simulink model "Filter_Model"  (R2020b)
settings: Solver=VariableStepAuto  StartTime=0.0  StopTime=10.0  RelTol=1e-3
settings Model: Creator=BIDITA PAUL  LastModifiedBy=BIDITA PAUL

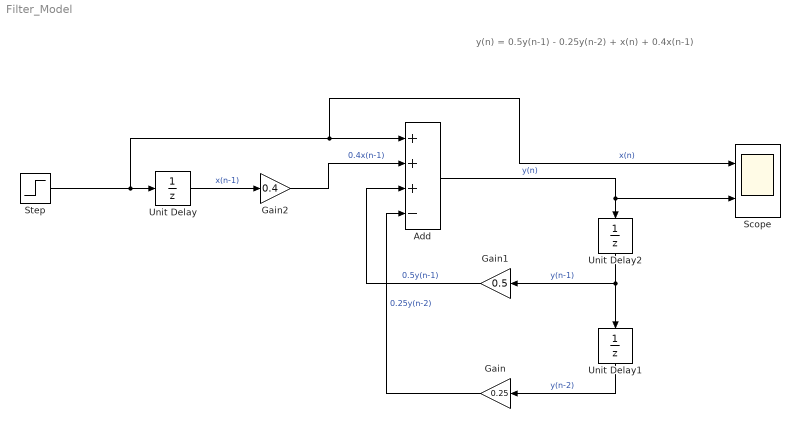
== system Filter_Model ==
  note: y(n) = 0.5y(n-1) - 0.25y(n-2) + x(n) + 0.4x(n-1)
  Add : Sum  Inputs=+++-
  Gain : Gain  Gain=0.25
  Gain1 : Gain  Gain=0.5
  Gain2 : Gain  Gain=0.4
  Scope : Scope  NumInputPorts=2
  Step : Step  SampleTime=0
  Unit Delay : UnitDelay  SampleTime=-1  HasFrameUpgradeWarning=on
  Unit Delay1 : UnitDelay  SampleTime=-1  HasFrameUpgradeWarning=on
  Unit Delay2 : UnitDelay  SampleTime=-1  HasFrameUpgradeWarning=on
  wires:
  Step/1 -> Add/1, Scope/1, Unit Delay/1  "x(n)"
  Unit Delay/1 -> Gain2/1  "x(n-1)"
  Add/1 -> Unit Delay2/1, Scope/2  "y(n)"
  Unit Delay2/1 -> Unit Delay1/1, Gain1/1  "y(n-1)"
  Unit Delay1/1 -> Gain/1  "y(n-2)"
  Gain/1 -> Add/4  "0.25y(n-2)"
  Gain1/1 -> Add/3  "0.5y(n-1)"
  Gain2/1 -> Add/2  "0.4x(n-1)"
